simulink library "TunableDelay"  (R2022b)
settings: Solver=VariableStepAuto  StartTime=0.0  StopTime=10.0  RelTol=1e-3
libraries: TunableDelayBtc x4
settings Model: Creator=ud1041536  LastModifiedBy=kl13806
settings SolverCC: AlgebraicLoopSolver=TrustRegion
settings DebuggingCC: UnconnectedInputMsg=warning  UnconnectedOutputMsg=warning  UnconnectedLineMsg=warning  SFMachineParentedDataDiag=warning  ArithmeticOperatorsInVariantConditions=warning
settings ModelReferenceCC: EnableRefExpFcnMdlSchedulingChecks=on
settings SFSimCC: SimUseLocalCustomCode=off  CustomCodeUndefinedFunction=UseInterfaceOnly
settings RTWCC: RTWUseLocalCustomCode=off  DLArmComputeVersion=19.05

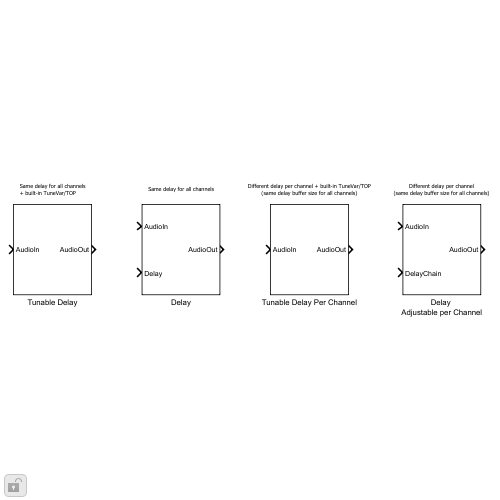
[thumbnail: Simulink's stored preview of the top-level diagram]
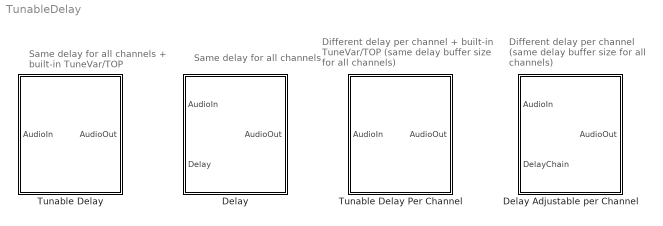
== system TunableDelay ==
  note: Same delay for all channels
      | + built-in TuneVar/TOP
  note: Same delay for all channels
  note: Different delay per channel + built-in TuneVar/TOP
      | (same delay buffer size for all channels)
  note: Different delay per channel
      | (same delay buffer size for all channels)
  Delay : Subsystem  mask(Fixed Alignment Delay){maxDelayTime=512, frameSize=32, numChannels=2, bufferAlias=[], headerFilename=[]}
      mask prompts: maxDelayTime "Max delay"; frameSize "Frame size"; numChannels "Num channels"; bufferAlias "Buffer alias"; headerFilename "Header file name"
      mask help:
      | This block takes two inputs - delay amount in samples and audio. The same input delay amount is applied to all channels.
      |
      | Note: Please provide a Buffer Alias to the delay in order to access and edit the Header File Name.
      |
      | SHARC+ circular buffer CRL only works for delay amount of type 'int32'.
      mask init:
      | blkh = gcbh;
      | % Copy discrete mask parameters into a classdef object
      | InnerLinkConfig = DelayConfig;
      | InnerLinkConfig.MaxDelayTime = maxDelayTime;
      | InnerLinkConfig.FrameSize = frameSize;
      | InnerLinkConfig.NumChannels = numChannels;
      | InnerLinkConfig.BufferAlias = bufferAlias;
      | InnerLinkConfig.HeaderFilename = headerFilename;
      mask Help:
      | Help on Mask Parameters:
      | 
      | Max Delay (in samples), Frame Size and Number of Channels help determine the circular buffer size. Buffer Alias and Header File Name are useful for memory management in cases where multiple delays are implemented. Both Buffer Alias and Header File Name are reflected in generated code.
      | 
      | Max Delay (in samples): Maximum delay that could be applied to the incoming audio.
      | Frame Size: Frame Size of the incoming audio
      | Number of Channels: Number of channels in incoming audio
      | Buffer Alias: Alias for the circular buffer allocated for this delay instance.
      | Header File Name: Name for header file that specifically manages the delays
      mask Callback bufferAlias:
      | % Get the mask parameter values. This is a cell
      | % array of character vectors.
      | maskStr = get_param(gcb,'bufferAlias');
      | 
      | % Check the value of 'bufferalias'
      | if ~(strcmp(maskStr,"[]"))
      |     % Set the visibility of all parameters on when
      |     set_param(gcb,'MaskVisibilities',{'on';'on';'on';'on';'on'});
      | else
      |     % Turn off the visibility of the 'headerfilename' field
      |     set_param(gcb,'MaskVisibilities',{'on';'on';'on';'on';'off'});
      | end
      | 
      | % Check if the 'bufferAlias' field is empty
      | if isempty(maskStr)
      |     % Turn off the visibility of the 'headerfilename' field
      |     set_param(gcb,'MaskVisibilities',{'on';'on';'on';'on';'off'});
      |     % Default the value of 'bufferAlias'
      |     set_param(gcb,'bufferAlias',"[]");
      | end
  Delay Adjustable per Channel : Subsystem  mask(Tunable Delay){maxDelayTime=512, frameSize=32, numChannels=2, bufferAlias=[], headerFilename=[]}
      mask prompts: maxDelayTime "Max delay"; frameSize "Frame size"; numChannels "Num channels"; bufferAlias "Buffer alias"; headerFilename "Header file name"
      mask help:
      | This block takes two inputs - delay amount in samples and audio. The input delay consists of individual delays for each channel.
      |
      | Note: Please provide a Buffer Alias to the delay in order to access and edit the Header File Name.
      |
      | SHARC+ circular buffer CRL only works for delay amount of type 'int32'.
      mask init:
      | blkh = gcbh;
      | % Copy discrete mask parameters into a classdef object
      | InnerLinkConfig = DelayPerChannelConfig;
      | InnerLinkConfig.MaxDelayTime = maxDelayTime;
      | InnerLinkConfig.FrameSize = frameSize;
      | InnerLinkConfig.NumChannels = numChannels;
      | InnerLinkConfig.BufferAlias = bufferAlias;
      | InnerLinkConfig.HeaderFilename = headerFilename;
      mask Help:
      | Help on Mask Parameters:
      | 
      | Max Delay (in samples), Frame Size and Number of Channels help determine the circular buffer size. Buffer Alias and Header File Name are useful for memory management in cases where multiple delays are implemented. Both Buffer Alias and Header File Name are reflected in generated code.
      | 
      | Max Delay (in samples): Maximum delay that could be applied to the incoming audio.
      | Frame Size: Frame Size of the incoming audio
      | Number of Channels: Number of channels in incoming audio
      | Buffer Alias: Alias for the circular buffer allocated for this delay instance.
      | Header File Name: Name for header file that specifically manages the delays
      | 
      | For example, if the incoming audio consists of three channels, the incoming delay should be a 1x3 matrix (e.g. [10 20 30]).
      | Each element of delay shall be applied to the corresponding channel fo incoming audio. In the above example, the first input channel would be delayed by 10 samples, the second channel by 20 samples and the third by 30 samples.
      mask Callback bufferAlias:
      | % Get the mask parameter values. This is a cell
      | % array of character vectors.
      | maskStr = get_param(gcb,'bufferAlias');
      | 
      | % Check the value of 'bufferalias'
      | if ~(strcmp(maskStr,"[]"))
      |     % Set the visibility of all parameters on when
      |     set_param(gcb,'MaskVisibilities',{'on';'on';'on';'on';'on'});
      | else
      |     % Turn off the visibility of the 'headerfilename' field
      |     set_param(gcb,'MaskVisibilities',{'on';'on';'on';'on';'off'});
      | end
      | 
      | % Check if the 'bufferAlias' field is empty
      | if isempty(maskStr)
      |     % Turn off the visibility of the 'headerfilename' field
      |     set_param(gcb,'MaskVisibilities',{'on';'on';'on';'on';'off'});
      |     % Default the value of 'bufferAlias'
      |     set_param(gcb,'bufferAlias',"[]");
      | end
  Tunable Delay : Subsystem  mask(Tunable Delay){MaskDelayType=In Milliseconds, FeatureName=Delay, MaskValue=[], maxDelayTime=512, frameSize=32, numChannels=2, bufferAlias=[], headerFilename=[]}
      mask prompts: MaskDelayType "Delay type"; FeatureName "Delay name/purpose"; MaskValue "Delay amount"; maxDelayTime "Max delay"; frameSize "Frame size"; numChannels "Num channels"; bufferAlias "Buffer alias"; headerFilename "Header file name"
      mask help:
      | This delay block delays the input by a specified amount in either samples or seconds. The same input delay amount is applied to all channels.
      |
      | Note: Please provide a Buffer Alias to the delay in order to access and edit the Header File Name.
      mask init:
      | blkh = gcbh;
      | % Copy discrete mask parameters into a classdef object
      | InnerLinkConfig = TunableDelayConfig;
      | InnerLinkConfig.DefaultDelayType = MaskDelayType;
      | InnerLinkConfig.DefaultDelayAmount = MaskValue;
      | InnerLinkConfig.MaxDelayTime = maxDelayTime;
      | InnerLinkConfig.FrameSize = frameSize;
      | InnerLinkConfig.NumChannels = numChannels;
      | InnerLinkConfig.BufferAlias = bufferAlias;
      | InnerLinkConfig.HeaderFilename = headerFilename;
      mask Help:
      | Help on Mask Parameters:
      | 
      | Max Delay (in samples), Frame Size and Number of Channels help determine the circular buffer size. Buffer Alias and Header File Name are useful for memory management in cases where multiple delays are implemented. Both Buffer Alias and Header File Name are reflected in generated code.
      | 
      | Max Delay (in samples): Maximum delay that could be applied to the incoming audio.
      | Frame Size: Frame Size of the incoming audio
      | Number of Channels: Number of channels in incoming audio
      | Buffer Alias: Alias for the circular buffer allocated for this delay instance.
      | Header File Name: Name for header file that specifically manages the delays
      mask TypeOptions MaskDelayType: In Samples | In Milliseconds
      mask TypeOptions FeatureName: InnerLink/FeatureName
      mask Callback bufferAlias:
      | % Get the mask parameter values. This is a cell
      | % array of character vectors.
      | maskStr = get_param(gcb,'bufferAlias');
      | 
      | % Check the value of 'bufferalias'
      | if ~(strcmp(maskStr,"[]"))
      |     % Set the visibility of all parameters on when
      |     set_param(gcb,'MaskVisibilities',{'on';'on';'on';'on';'on';'on';'on';'on'});
      | else
      |     % Turn off the visibility of the 'headerfilename' field
      |     set_param(gcb,'MaskVisibilities',{'on';'on';'on';'on';'on';'on';'on';'off'});
      | end
      | 
      | % Check if the 'bufferAlias' field is empty
      | if isempty(maskStr)
      |     % Turn off the visibility of the 'headerfilename' field
      |     set_param(gcb,'MaskVisibilities',{'on';'on';'on';'on';'on';'on';'on';'off'});
      |     % Default the value of 'bufferAlias'
      |     set_param(gcb,'bufferAlias',"[]");
      | end
  Tunable Delay Per Channel : Subsystem  mask(Tunable Delay){MaskDelayType=In Milliseconds, FeatureName=Delay, MaskValue=[], maxDelayTime=512, frameSize=32, numChannels=2, bufferAlias=[], headerFilename=[]}
      mask prompts: MaskDelayType "Delay type"; FeatureName "Delay name/purpose"; MaskValue "Delay amount"; maxDelayTime "Max delay"; frameSize "Frame size"; numChannels "Num channels"; bufferAlias "Buffer alias"; headerFilename "Header file name"
      mask help:
      | This delay block delays the input by a specified amount in either samples or seconds. The same input delay amount is applied to all channels.
      |
      | Note: Please provide a Buffer Alias to the delay in order to access and edit the Header File Name.
      mask init:
      | blkh = gcbh;
      | % Copy discrete mask parameters into a classdef object
      | InnerLinkConfig = TunableDelayPerChannelConfig;
      | InnerLinkConfig.DefaultDelayType = MaskDelayType;
      | InnerLinkConfig.DefaultDelayAmount = MaskValue;
      | InnerLinkConfig.MaxDelayTime = maxDelayTime;
      | InnerLinkConfig.FrameSize = frameSize;
      | InnerLinkConfig.NumChannels = numChannels;
      | InnerLinkConfig.BufferAlias = bufferAlias;
      | InnerLinkConfig.HeaderFilename = headerFilename;
      mask Help:
      | Help on Mask Parameters:
      | 
      | Max Delay (in samples), Frame Size and Number of Channels help determine the circular buffer size. Buffer Alias and Header File Name are useful for memory management in cases where multiple delays are implemented. Both Buffer Alias and Header File Name are reflected in generated code.
      | 
      | Max Delay (in samples): Maximum delay that could be applied to the incoming audio.
      | Frame Size: Frame Size of the incoming audio
      | Number of Channels: Number of channels in incoming audio
      | Buffer Alias: Alias for the circular buffer allocated for this delay instance.
      | Header File Name: Name for header file that specifically manages the delays
      mask TypeOptions MaskDelayType: In Samples | In Milliseconds
      mask TypeOptions FeatureName: InnerLink/FeatureName
      mask Callback bufferAlias:
      | % Get the mask parameter values. This is a cell
      | % array of character vectors.
      | maskStr = get_param(gcb,'bufferAlias');
      | 
      | % Check the value of 'bufferalias'
      | if ~(strcmp(maskStr,"[]"))
      |     % Set the visibility of all parameters on when
      |     set_param(gcb,'MaskVisibilities',{'on';'on';'on';'on';'on';'on';'on';'on'});
      | else
      |     % Turn off the visibility of the 'headerfilename' field
      |     set_param(gcb,'MaskVisibilities',{'on';'on';'on';'on';'on';'on';'on';'off'});
      | end
      | 
      | % Check if the 'bufferAlias' field is empty
      | if isempty(maskStr)
      |     % Turn off the visibility of the 'headerfilename' field
      |     set_param(gcb,'MaskVisibilities',{'on';'on';'on';'on';'on';'on';'on';'off'});
      |     % Default the value of 'bufferAlias'
      |     set_param(gcb,'bufferAlias',"[]");
      | end

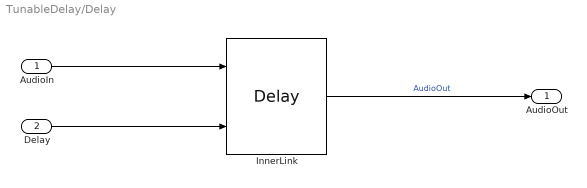
== system TunableDelay/Delay ==
  AudioIn : Inport
  Delay : Inport  Port=2
  InnerLink : TunableDelayBtc/Delay  Config=InnerLinkConfig
      settings: SourceProductName=Bose Blocklib
  AudioOut : Outport
  wires:
  InnerLink/1 -> AudioOut/1  "AudioOut"
  AudioIn/1 -> InnerLink/1
  Delay/1 -> InnerLink/2

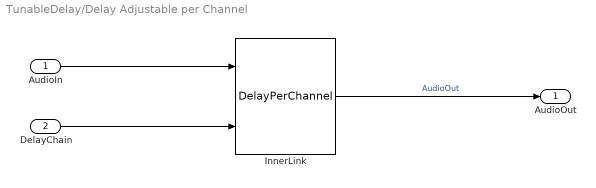
== system TunableDelay/Delay Adjustable per Channel ==
  AudioIn : Inport
  DelayChain : Inport  Port=2
  InnerLink : TunableDelayBtc/DelayPerChannel  Config=InnerLinkConfig
      settings: SourceProductName=Bose Blocklib
  AudioOut : Outport
  wires:
  InnerLink/1 -> AudioOut/1  "AudioOut"
  AudioIn/1 -> InnerLink/1
  DelayChain/1 -> InnerLink/2

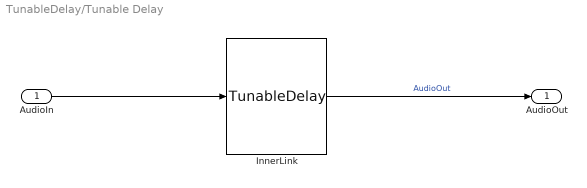
== system TunableDelay/Tunable Delay ==
  AudioIn : Inport
  InnerLink : TunableDelayBtc/TunableDelay  Config=InnerLinkConfig  FeatureName=Delay
      settings: SourceProductName=Bose Blocklib
  AudioOut : Outport
  wires:
  InnerLink/1 -> AudioOut/1  "AudioOut"
  AudioIn/1 -> InnerLink/1

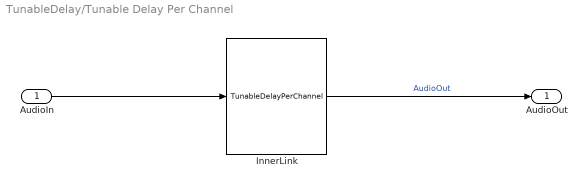
== system TunableDelay/Tunable Delay Per Channel ==
  AudioIn : Inport
  InnerLink : TunableDelayBtc/TunableDelayPerChannel  Config=InnerLinkConfig  FeatureName=Delay
      settings: SourceProductName=Bose Blocklib
  AudioOut : Outport
  wires:
  InnerLink/1 -> AudioOut/1  "AudioOut"
  AudioIn/1 -> InnerLink/1
